simulink model "kkadai21"  (R2021b)
settings: Solver=VariableStepAuto  StartTime=0.0  StopTime=800  RelTol=1e-3
settings Model: Creator=is221042  LastModifiedBy=is221042

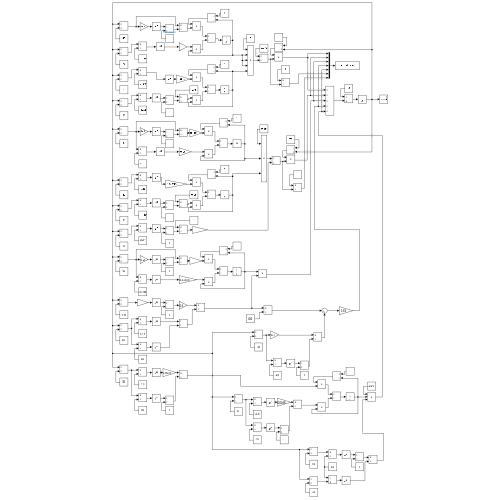
[thumbnail: Simulink's stored preview of the top-level diagram]
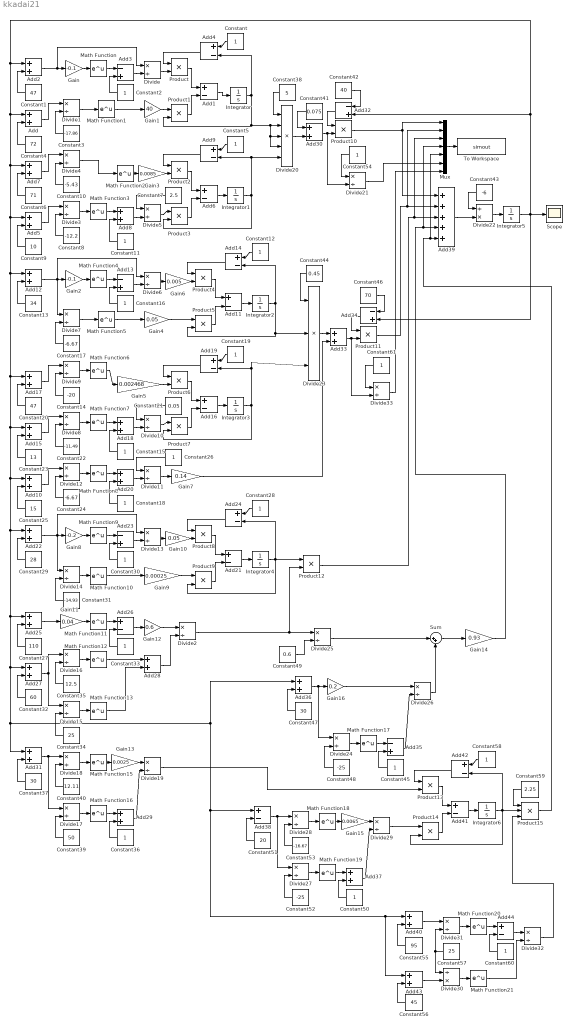
== system kkadai21 ==
  Add{,2,5,7..8,10,12,15,17..18,20,22,25,27..31,33,36..37,40,43} (23 alike) : Sum
  Add{1,4,6,9,11,14,16,19,21,24,26,38,41..42,44} (15 alike) : Sum  Inputs=+-
  Add{3,13,23,32,34..35} (6 alike) : Sum  Inputs=-+
  Add39 : Sum  Inputs=+++++
  Constant{,2,5,11..12,15..16,18..19,26,28,30,33,36,45,50,54,58,60..61} (20 alike) : Constant
  Constant1 : Constant  Value=47
  Constant10 : Constant  Value=-5.43
  Constant13 : Constant  Value=34
  Constant14 : Constant  Value=-20
  Constant17 : Constant  Value=-6.67
  Constant20 : Constant  Value=47
  Constant21 : Constant  Value=0.05
  Constant22 : Constant  Value=-11.49
  Constant23 : Constant  Value=13
  Constant24 : Constant  Value=-6.67
  Constant25 : Constant  Value=15
  Constant27 : Constant  Value=110
  Constant29 : Constant  Value=28
  Constant3 : Constant  Value=-17.86
  Constant31 : Constant  Value=-14.93
  Constant32 : Constant  Value=60
  Constant34 : Constant  Value=25
  Constant35 : Constant  Value=12.5
  Constant37 : Constant  Value=30
  Constant38 : Constant  Value=5
  Constant39 : Constant  Value=50
  Constant4 : Constant  Value=72
  Constant40 : Constant  Value=12.11
  Constant41 : Constant  Value=0.075
  Constant42 : Constant  Value=40
  Constant43 : Constant  Value=-6
  Constant44 : Constant  Value=0.45
  Constant46 : Constant  Value=70
  Constant47 : Constant  Value=30
  Constant48 : Constant  Value=-25
  Constant49 : Constant  Value=0.6
  Constant51 : Constant  Value=20
  Constant52 : Constant  Value=-25
  Constant53 : Constant  Value=-16.67
  Constant55 : Constant  Value=95
  Constant56 : Constant  Value=45
  Constant57 : Constant  Value=25
  Constant59 : Constant  Value=2.25
  Constant6 : Constant  Value=71
  Constant7 : Constant  Value=2.5
  Constant8 : Constant  Value=-12.2
  Constant9 : Constant  Value=10
  Divide{,1..19,21,24..29,31..33} (30 alike) : Product  Inputs=*/
  Divide20 : Product  Inputs=*****
  Divide22 : Product  Inputs=/*
  Divide23 : Product  Inputs=***
  Divide30 : Product  Inputs=/*
  Gain : Gain  Gain=-0.1
  Gain1 : Gain  Gain=40
  Gain10 : Gain  Gain=0.05
  Gain11 : Gain  Gain=0.04
  Gain12 : Gain  Gain=0.6
  Gain13 : Gain  Gain=0.0025
  Gain14 : Gain  Gain=0.93
  Gain15 : Gain  Gain=0.0065
  Gain16 : Gain  Gain=0.2
  Gain2 : Gain  Gain=-0.1
  Gain3 : Gain  Gain=0.0085
  Gain4 : Gain  Gain=0.05
  Gain5 : Gain  Gain=0.002468
  Gain6 : Gain  Gain=0.005
  Gain7 : Gain  Gain=0.14
  Gain8 : Gain  Gain=-0.2
  Gain9 : Gain  Gain=0.00025
  Integrator : Integrator  InitialCondition=0.17016
  Integrator1 : Integrator  InitialCondition=0.02520
  Integrator2 : Integrator  InitialCondition=0.00318
  Integrator3 : Integrator  InitialCondition=0.26486
  Integrator4 : Integrator  InitialCondition=0.89877
  Integrator5 : Integrator  InitialCondition=-61.3
  Integrator6 : Integrator  InitialCondition=0.05037
  Math Function{,1..13,15..21} (21 alike) : Math  SaturateOnIntegerOverflow=on
  Mux : Mux  Inputs=7
  Product{,1..14} (15 alike) : Product
  Product15 : Product  Inputs=3
  Scope : Scope
  Sum : Sum  Inputs=|++
  To Workspace : ToWorkspace  VariableName=simout  SaveFormat=Timeseries  SampleTime=-1
  wires:
  Add2/1 -> Divide/1, Gain/1
  Constant1/1 -> Add2/2
  Gain/1 -> Math Function/1
  Math Function/1 -> Add3/1
  Add3/1 -> Divide/2
  Constant2/1 -> Add3/2
  Divide/1 -> Product/2
  Product/1 -> Add1/1
  Product1/1 -> Add1/2
  Gain1/1 -> Product1/1
  Math Function1/1 -> Gain1/1
  Divide1/1 -> Math Function1/1
  Constant3/1 -> Divide1/2
  Constant4/1 -> Add/2
  Add/1 -> Divide1/1
  Add1/1 -> Integrator/1
  Integrator/1 -> Add4/2, Product1/2, Divide20/2, Divide20/4, Divide20/3
  Add4/1 -> Product/1
  Constant/1 -> Add4/1
  Product2/1 -> Add6/1
  Constant5/1 -> Add9/1
  Add5/1 -> Divide3/1
  Constant9/1 -> Add5/2
  Constant8/1 -> Divide3/2
  Add9/1 -> Product2/1
  Constant6/1 -> Add7/2
  Math Function2/1 -> Gain3/1
  Product3/1 -> Add6/2
  Divide3/1 -> Math Function3/1
  Integrator1/1 -> Divide20/5, Add9/2, Product3/2
  Add6/1 -> Integrator1/1
  Gain3/1 -> Product2/2
  Constant10/1 -> Divide4/2
  Divide4/1 -> Math Function2/1
  Add7/1 -> Divide4/1
  Math Function3/1 -> Add8/1
  Constant11/1 -> Add8/2
  Divide5/1 -> Product3/1
  Add8/1 -> Divide5/2
  Constant7/1 -> Divide5/1
  Product4/1 -> Add11/1
  Constant14/1 -> Divide9/2
  Add18/1 -> Divide10/2
  Constant12/1 -> Add14/1
  Constant17/1 -> Divide7/2
  Add17/1 -> Divide9/1
  Add14/1 -> Product4/1
  Math Function5/1 -> Gain4/1
  Constant16/1 -> Add13/2
  Constant13/1 -> Add12/2
  Gain4/1 -> Product5/1
  Add16/1 -> Integrator3/1
  Integrator3/1 -> Add19/2, Divide23/3, Product7/2
  Divide8/1 -> Math Function7/1
  Math Function4/1 -> Add13/1
  Add19/1 -> Product6/1
  Constant23/1 -> Add15/2
  Product7/1 -> Add16/2
  Gain5/1 -> Product6/2
  Constant22/1 -> Divide8/2
  Math Function7/1 -> Add18/1
  Constant19/1 -> Add19/1
  Divide9/1 -> Math Function6/1
  Add15/1 -> Divide8/1
  Product6/1 -> Add16/1
  Constant15/1 -> Add18/2
  Constant21/1 -> Divide10/1
  Divide10/1 -> Product7/1
  Product5/1 -> Add11/2
  Divide7/1 -> Math Function5/1
  Math Function6/1 -> Gain5/1
  Constant20/1 -> Add17/2
  Add12/1 -> Divide7/1, Divide6/1, Gain2/1
  Integrator2/1 -> Add14/2, Product5/2, Divide23/2
  Add13/1 -> Divide6/2
  Gain2/1 -> Math Function4/1
  Add11/1 -> Integrator2/1
  Divide6/1 -> Gain6/1
  Gain6/1 -> Product4/2
  Constant18/1 -> Add20/2
  Constant26/1 -> Divide11/1
  Add10/1 -> Divide12/1
  Constant25/1 -> Add10/2
  Constant24/1 -> Divide12/2
  Divide12/1 -> Math Function8/1
  Math Function8/1 -> Add20/1
  Add20/1 -> Divide11/2
  Divide11/1 -> Gain7/1
  Divide13/1 -> Gain10/1
  Gain10/1 -> Product8/2
  Add21/1 -> Integrator4/1
  Add23/1 -> Divide13/2
  Gain8/1 -> Math Function9/1
  Integrator4/1 -> Product12/1, Add24/2, Product9/2
  Add22/1 -> Divide14/1, Divide13/1, Gain8/1
  Divide14/1 -> Math Function10/1
  Math Function9/1 -> Add23/1
  Math Function10/1 -> Gain9/1
  Constant30/1 -> Add23/2
  Constant29/1 -> Add22/2
  Product8/1 -> Add21/1
  Gain9/1 -> Product9/1
  Product9/1 -> Add21/2
  Constant31/1 -> Divide14/2
  Constant28/1 -> Add24/1
  Add24/1 -> Product8/1
  Constant27/1 -> Add25/2
  Add25/1 -> Gain11/1
  Gain11/1 -> Math Function11/1
  Constant33/1 -> Add26/2
  Math Function11/1 -> Add26/1
  Add26/1 -> Gain12/1
  Constant32/1 -> Add27/2
  Constant34/1 -> Divide15/2
  Constant35/1 -> Divide16/2
  Add27/1 -> Divide15/1, Divide16/1
  Divide16/1 -> Math Function12/1
  Divide15/1 -> Math Function13/1
  Math Function12/1 -> Add28/1
  Math Function13/1 -> Add28/2
  Divide17/1 -> Math Function16/1
  Add31/1 -> Divide17/1, Divide18/1
  Constant39/1 -> Divide17/2
  Divide18/1 -> Math Function15/1
  Constant37/1 -> Add31/2
  Constant40/1 -> Divide18/2
  Math Function15/1 -> Gain13/1
  Gain13/1 -> Divide19/1
  Math Function16/1 -> Add29/1
  Constant36/1 -> Add29/2
  Add29/1 -> Divide19/2
  Constant38/1 -> Divide20/1
  Divide20/1 -> Add30/2
  Constant41/1 -> Add30/1
  Add30/1 -> Divide21/2, Product10/2
  Integrator5/1 -> Add32/2, Add2/1, Add/1, Add7/1, Add5/1, Add12/1, Add31/1, Add43/1, Add40/1, Add38/1, Add36/1, Add27/1, Add25/1, Add22/1, Add10/1, Add15/1, Add17/1, Add34/2, Scope/1
  Constant42/1 -> Add32/1
  Add32/1 -> Product10/1
  Product10/1 -> Mux/1, Add39/1
  Add39/1 -> Divide22/2
  Constant43/1 -> Divide22/1
  Divide22/1 -> Integrator5/1
  Constant44/1 -> Divide23/1
  Add34/1 -> Product11/1
  Constant46/1 -> Add34/1
  Divide23/1 -> Add33/1
  Product11/1 -> Mux/2, Add39/2
  Gain7/1 -> Add33/2
  Gain12/1 -> Divide2/1
  Add28/1 -> Divide2/2
  Divide2/1 -> Divide25/1, Product12/2
  Product12/1 -> Mux/3, Add39/3
  Constant47/1 -> Add36/2
  Add36/1 -> Gain16/1, Divide24/1
  Divide24/1 -> Math Function17/1
  Add35/1 -> Divide26/2
  Constant45/1 -> Add35/2
  Gain16/1 -> Divide26/1
  Math Function17/1 -> Add35/1
  Constant48/1 -> Divide24/2
  Constant51/1 -> Add38/2
  Constant53/1 -> Divide28/2
  Divide28/1 -> Math Function18/1
  Add38/1 -> Divide27/1, Divide28/1
  Divide27/1 -> Math Function19/1
  Add37/1 -> Divide29/2
  Constant50/1 -> Add37/2
  Math Function18/1 -> Gain15/1
  Gain15/1 -> Divide29/1
  Math Function19/1 -> Add37/1
  Constant52/1 -> Divide27/2
  Constant55/1 -> Add40/2
  Constant57/1 -> Divide30/1, Divide31/2
  Divide31/1 -> Math Function20/1
  Add40/1 -> Divide31/1
  Divide30/1 -> Math Function21/1
  Math Function21/1 -> Divide32/2
  Math Function20/1 -> Add44/1
  Add44/1 -> Divide32/1
  Integrator6/1 -> Add42/2, Product15/2, Product14/2
  Product13/1 -> Add41/1
  Product14/1 -> Add41/2
  Constant58/1 -> Add42/1
  Divide29/1 -> Product14/1
  Add42/1 -> Product13/1
  Add41/1 -> Integrator6/1
  Divide19/1 -> Product13/2
  Constant59/1 -> Product15/1
  Add43/1 -> Divide30/2
  Constant56/1 -> Add43/2
  Constant60/1 -> Add44/2
  Divide32/1 -> Product15/3
  Constant49/1 -> Divide25/2
  Divide25/1 -> Sum/1
  Sum/1 -> Gain14/1
  Divide26/1 -> Sum/2
  Gain14/1 -> Mux/4, Add39/4
  Product15/1 -> Mux/5, Add39/5
  Mux/1 -> To Workspace/1
  Constant54/1 -> Divide21/1
  Constant61/1 -> Divide33/1
  Add33/1 -> Divide33/2, Product11/2
  Divide21/1 -> Mux/6
  Divide33/1 -> Mux/7
